simulink model "callZumoExtrinsic"  (R2014a)
settings: Solver=FixedStepDiscrete  StartTime=0.0  StopTime=inf  FixedStep=0.1  RelTol=1e-3
libraries: simulink x1
settings Model: Creator=nrattner  LastModifiedBy=nrattner

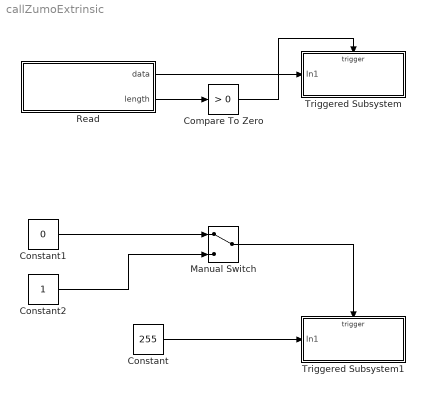
== system callZumoExtrinsic ==
  Compare To Zero : simulink/Logic and Bit Operations/Compare To Zero  relop=>  OutDataTypeStr=boolean
  Constant : Constant  Value=255
  Constant1 : Constant  Value=0
  Constant2 : Constant
  Manual Switch : ManualSwitch
  Read : MATLAB Function  TreatAsAtomicUnit=on
  Triggered Subsystem : Subsystem  TreatAsAtomicUnit=on
  Triggered Subsystem1 : Subsystem  TreatAsAtomicUnit=on
  wires:
  Read/1(data) -> Triggered Subsystem/1(In1)
  Read/2(length) -> Compare To Zero/1
  Compare To Zero/1 -> Triggered Subsystem/Trigger
  Constant/1 -> Triggered Subsystem1/1(In1)
  Manual Switch/1 -> Triggered Subsystem1/Trigger
  Constant2/1 -> Manual Switch/2
  Constant1/1 -> Manual Switch/1

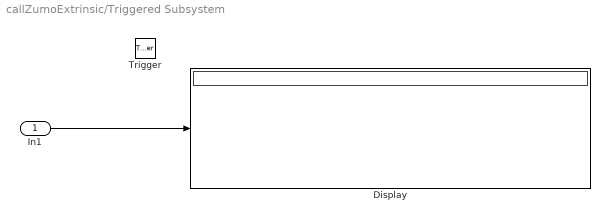
== system callZumoExtrinsic/Triggered Subsystem ==
  In1 : Inport
  Trigger : TriggerPort
  Display : Display
  wires:
  In1/1 -> Display/1

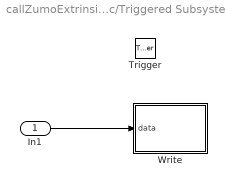
== system callZumoExtrinsic/Triggered Subsystem1 ==
  In1 : Inport
  Trigger : TriggerPort
  Write : MATLAB Function  TreatAsAtomicUnit=on
  wires:
  In1/1 -> Write/1(data)

== matlab function callZumoExtrinsic/Triggered Subsystem1/Write ==
  data: data input
function write(data)
%#codegen

coder.extrinsic('comms.writeZumoBluetooth')
comms.writeZumoBluetooth(data);

== matlab function callZumoExtrinsic/Read ==
  data: data output; length output
function [data, length] = read()
%#codegen

coder.extrinsic('comms.readZumoBluetooth');

data = uint8(0);
length = 0;
[length, data] = comms.readZumoBluetooth();

end
